simulink model "EM_Model"  (R2017b)
settings: Solver=ode45  StartTime=0.0  StopTime=10.0  RelTol=1e-3
undefined symbols (not defined in the file): k1, k2, k3, Ki, Ks, L, m1, m2, m3, R, u0, x0
settings Model: Creator=lasse  LastModifiedBy=lasse

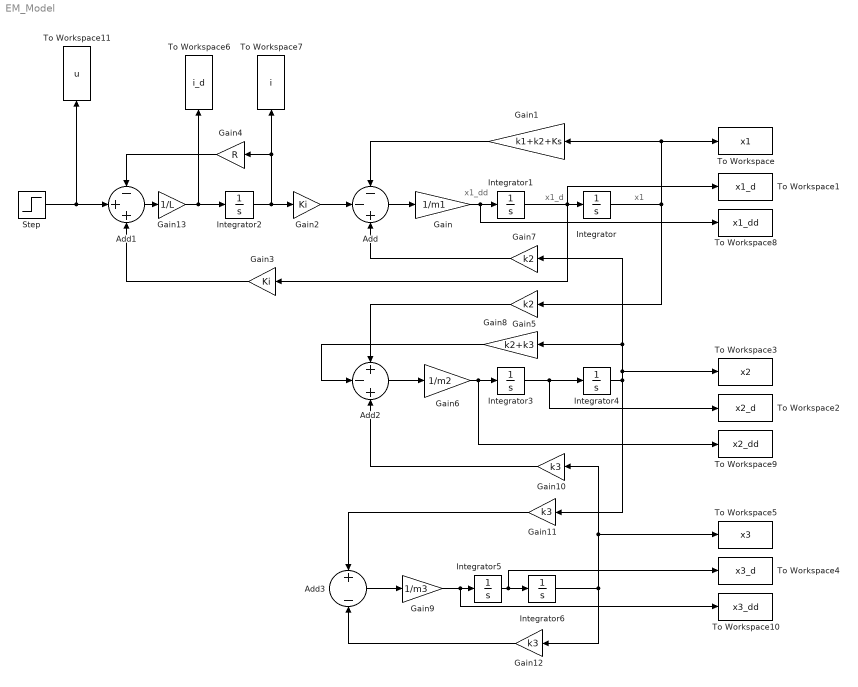
== system EM_Model ==
  note: x1
  note: x1_d
  note: x1_dd
  Add : Sum  Inputs=--+
  Add1 : Sum  Inputs=-++
  Add2 : Sum  Inputs=+-+
  Add3 : Sum  Inputs=+-
  Gain : Gain  Gain=1/m1
  Gain1 : Gain  Gain=k1+k2+Ks
  Gain10 : Gain  Gain=k3
  Gain11 : Gain  Gain=k3
  Gain12 : Gain  Gain=k3
  Gain13 : Gain  Gain=1/L
  Gain2 : Gain  Gain=Ki
  Gain3 : Gain  Gain=Ki
  Gain4 : Gain  Gain=R
  Gain5 : Gain  Gain=k2
  Gain6 : Gain  Gain=1/m2
  Gain7 : Gain  Gain=k2
  Gain8 : Gain  Gain=k2+k3
  Gain9 : Gain  Gain=1/m3
  Integrator : Integrator  InitialCondition=x0(3)
  Integrator1 : Integrator  InitialCondition=x0(2)
  Integrator2 : Integrator  InitialCondition=x0(1)
  Integrator3 : Integrator  InitialCondition=x0(4)
  Integrator4 : Integrator  InitialCondition=x0(5)
  Integrator5 : Integrator  InitialCondition=x0(6)
  Integrator6 : Integrator  InitialCondition=x0(7)
  Step : Step  After=u0  SampleTime=0
  To Workspace : ToWorkspace  VariableName=x1  SaveFormat=Structure With Time  SampleTime=-1
  To Workspace1 : ToWorkspace  VariableName=x1_d  SaveFormat=Structure With Time  SampleTime=-1
  To Workspace10 : ToWorkspace  VariableName=x3_dd  SaveFormat=Structure With Time  SampleTime=-1
  To Workspace11 : ToWorkspace  VariableName=u  SaveFormat=Structure With Time  SampleTime=-1
  To Workspace2 : ToWorkspace  VariableName=x2_d  SaveFormat=Structure With Time  SampleTime=-1
  To Workspace3 : ToWorkspace  VariableName=x2  SaveFormat=Structure With Time  SampleTime=-1
  To Workspace4 : ToWorkspace  VariableName=x3_d  SaveFormat=Structure With Time  SampleTime=-1
  To Workspace5 : ToWorkspace  VariableName=x3  SaveFormat=Structure With Time  SampleTime=-1
  To Workspace6 : ToWorkspace  VariableName=i_d  SaveFormat=Structure With Time  SampleTime=-1
  To Workspace7 : ToWorkspace  VariableName=i  SaveFormat=Structure With Time  SampleTime=-1
  To Workspace8 : ToWorkspace  VariableName=x1_dd  SaveFormat=Structure With Time  SampleTime=-1
  To Workspace9 : ToWorkspace  VariableName=x2_dd  SaveFormat=Structure With Time  SampleTime=-1
  wires:
  Integrator1/1 -> Gain3/1, To Workspace1/1, Integrator/1
  Gain/1 -> To Workspace8/1, Integrator1/1
  Add/1 -> Gain/1
  Gain1/1 -> Add/1
  Integrator/1 -> To Workspace/1, Gain1/1, Gain5/1
  Gain2/1 -> Add/2
  Integrator2/1 -> Gain4/1, To Workspace7/1, Gain2/1
  Gain3/1 -> Add1/3
  Gain4/1 -> Add1/1
  Integrator3/1 -> To Workspace2/1, Integrator4/1
  Gain6/1 -> To Workspace9/1, Integrator3/1
  Gain5/1 -> Add2/1
  Add2/1 -> Gain6/1
  Integrator4/1 -> Gain11/1, Gain8/1, Gain7/1, To Workspace3/1
  Gain7/1 -> Add/3
  Gain8/1 -> Add2/2
  Integrator5/1 -> Integrator6/1, To Workspace4/1
  Gain9/1 -> To Workspace10/1, Integrator5/1
  Integrator6/1 -> Gain10/1, To Workspace5/1, Gain12/1
  Gain10/1 -> Add2/3
  Add3/1 -> Gain9/1
  Gain11/1 -> Add3/1
  Gain12/1 -> Add3/2
  Step/1 -> Add1/2, To Workspace11/1
  Gain13/1 -> Integrator2/1, To Workspace6/1
  Add1/1 -> Gain13/1
